simulink model "SDRE_MPTA_SDRE_newMODEL"  (R2024a)
settings: Solver=ode23t  StartTime=0  StopTime=27.8  RelTol=1e-3
values from neighbouring files (symbols this model uses):
  B = 0.002277    [initial_value.m]
  coef = readmatrix(ReadPath_coef)    [inital.m]
  command_t = readmatrix(ReadPath_command_t)    [inital.m]
  J = 0.00782    [initial_value.m]
  Lambda_m = 0.30175    [initial_value.m]
  Ld = 18e-3    (= 0.018)    [initial_value.m]
  Ldq = Ld - Lq    [inital.m]
  Lq = 32e-3    (= 0.032)    [initial_value.m]
  Polepairs = 3    [initial_value.m]
  rate1 = 3    [inital.m]
  rate2 = 1    [inital.m]
  Rs = 2.5    [initial_value.m]
  timestep = 1e-5    (= 1e-05)    [inital.m]
  V = [V_11 V_12;V_21 V_22]    [Create_MVG.m]
undefined symbols (not defined in the file or in its folder): rate
libraries: spsControlledVoltageSourceLib x6, spsPermanentMagnetSynchronousMachineLib x2, spsGroundLib x2, sps_lib x1
(part 2 of 2)

== matlab function SDRE_MPTA_SDRE_newMODEL/nomal3/toq to voltageABC6/MATLAB Function1 ==
  data: velo_fb input; id_fb input; iq_fb input; velo_ref input; id_ref input; iq_ref input; ud output; uq output; ud1 output; uq1 output; id_dot input; iq_dot input; ud2 output; uq2 output; velo_error output; id_error output; iq_error output
function [ud,uq,ud1,uq1,ud2,uq2,velo_error,id_error,iq_error] = SDRE_motor(velo_fb,id_fb,iq_fb,velo_ref,id_ref,iq_ref,id_dot,iq_dot)

ud = zeros(1, 1, 'double');
uq = zeros(1, 1, 'double');

%change data from [1*1] to singal input
Q = zeros(3, 3, 'double');

if isempty(id_dot)
    id_dot=0;
    iq_dot=0;
end


% velo_error   = 0;
% id_error     = 0;
% iq_error     = 0;

velo_error   = velo_fb   - velo_ref;
id_error     = id_fb     - id_ref;
iq_error     = iq_fb     - iq_ref;

if isempty(iq_error)
    velo_error=0;
    id_error=0;
    iq_error =0;
end

error = [velo_error iq_error id_error];

[Ld,Lq,Rs,Lambda_m,Polepairs,J,B]  = initial_value;
Ldq = Ld-Lq;

% A11 = -B/J; A12 = 3*Polepairs^2 *Lambda_m/(8*J); A13 = 3*Polepairs^2 *Ldq*iq_error/(8*J);
% A21 = -Lambda_m/(Lq) - Ld*id_error/(2*Lq); A22 = -Rs/Lq; A23 = - Ld*velo_error/(2*Lq);
% A31 = Lq*iq_error/(2*Ld); A32 =Lq*velo_error/(2*Ld); A33 = -Rs/Ld;

% A11 = -B/J; A12 = 3*Polepairs^2 *Lambda_m/(4*J); A13 = 3*Polepairs^2 *Ldq*iq_error/(4*J);
% A21 = -Lambda_m/(Lq) - Ld*id_error/(Lq); A22 = -Rs/Lq; A23 = 0;
% A31 = Lq*iq_error/(Ld); A32 =0; A33 = -Rs/Ld;
% 
% B11 = 0;B12 =0;
% B21=1/Lq;B22=0;
% B31=0;B32=1/Ld;

A11 = -B*Polepairs/J; A12 = 3*Polepairs^2 *(Lambda_m + Ldq*id_ref)/(2*J); A13 = 3*Polepairs^2 *Ldq*iq_fb/(2*J);
A21 = (-Lambda_m-Ld*id_fb)/(Lq) - Ld*id_error/(Lq); A22 = -Rs/Lq; A23 = -Ld*velo_ref/Lq;
A31 = Lq*iq_fb/(Ld); A32 =Lq*velo_ref/Ld; A33 = -Rs/Ld;

B11 = 0;B12 =0;
B21=1/Lq;B22=0;
B31=0;B32=1/Ld;


A = [A11 A12 A13 ;
     A21 A22 A23 ;
     A31 A32 A33];

B = [B11 B12;
     B21 B22;
     B31 B32];


rate = sqrt(iq_error^2 + id_error^2);
Q=diag([5000 1+exp(-rate) 10000+exp(-rate)]);
%Q=diag([800 1+exp(-rate) 100+exp(-rate)]);
R=diag([1 1]);

[P_ss_care,~]=SDA_CARE(A,B,Q,R);


% ucq = Rs*iq_ref + Lq*iq_dot + velo_ref*(Ld*id_ref+Lambda_m);
% ucd = Rs*id_ref + Ld*id_dot - velo_ref*Lq*iq_ref;


ucq = Rs*iq_ref + Lambda_m*velo_ref + Lq*iq_dot + Ld*id_error*velo_ref + Ld*velo_fb*id_ref;
ucd = Rs*id_ref + Ld*id_dot - Lq*iq_error*velo_ref - Lq*velo_fb*iq_ref;
if ucq > 1e5
    ucq =0;
end

if ucd > 1e5
    ucd =0;
end

u_redeem = -inv(R)*B'*P_ss_care*error';

% uq =  ucq ;
% ud =  ucd ;

uq =  ucq + u_redeem(1) ;
ud =  ucd + u_redeem(2) ;

ud1 = ucd ;
uq1 = ucq;

ud2 = u_redeem(2) ;
uq2 = u_redeem(1) ;


ud = (reshape(ud, 1, 1));
uq = (reshape(uq, 1, 1));


end

== matlab function SDRE_MPTA_SDRE_newMODEL/SDRE1 ==
  data: output_u1 output; Velocity1_ref output; T_load_1 output; Theta1_fb input; Velocity1_fb input; Acc1_fb input; Theta1_ref input; Theta3_ref input; Velocity1_ref input; Velocity3_ref input; Acc1_ref input; Acc3_ref input; output_u2 output; Velocity3_ref output; T_load_2 output; Theta3_fb input; Velocity3_fb input; Acc3_fb input; time input
function [output_u1,Velocity1_ref,T_load_1,output_u2,Velocity3_ref,T_load_2] = Robots_state(Theta1_fb,Velocity1_fb,Acc1_fb,Theta1_ref,Theta3_ref,Velocity1_ref,Velocity3_ref,Acc1_ref,Acc3_ref, Theta3_fb,  Velocity3_fb,Acc3_fb,time)
    %change data from [1*1] to singal input
    Acc3_ref = reshape(Acc3_ref, 1, []);

    Theta1_error =Theta1_fb - Theta1_ref;
    Velocity1_error = Velocity1_fb - Velocity1_ref;
    Acc1_error = Acc1_ref - Acc1_fb;

    Theta3_error = Theta3_fb - Theta3_ref;    
    Velocity3_error = Velocity3_fb - Velocity3_ref;
    Acc3_error = Acc3_ref - Acc3_fb;

    
    Acc_ref = [Acc1_ref;Acc3_ref];
    Velo_ref = [Velocity1_ref;Velocity3_ref];
    Theta_ref = [Theta1_ref;Theta3_ref];
    error_robot = [Theta1_error Theta3_error Velocity1_error Velocity3_error 0];

    Q=diag([10 10 1000 1000 0]);
    R=diag([1 1]);

    zeta = exp(-5*time);

    [M_fb,V_fb,G_sd_fb]=Create_MVG(Theta1_fb,Theta3_fb,Velocity1_fb,Velocity3_fb);
    [M_ref,V_ref,G_sd_ref]=Create_MVG(Theta1_ref,Theta3_ref,Velocity1_ref,Velocity3_ref);
    gf = M_fb*Acc_ref - M_ref*Acc_ref + V_fb*Velo_ref - V_ref*Velo_ref + G_sd_fb*Theta_ref - G_sd_ref*Theta_ref;
    A11 = zeros(2);
    A12 = eye(2);
    A13 = [0;0];
    A21 = -(M_fb)\G_sd_fb;
    A22 = -(M_fb)\V_fb;
    A23 = -((M_fb)\gf)/zeta;
    A31 = [0 0];
    A32 = [0 0];
    A33 = -5;
    A = [A11 A12 A13;A21 A22 A23;A31 A32 A33];
    B1 = zeros(2);
    B2 = inv(M_fb);
    B = [B1;B2;0 0];

    [P_ss_care,~]=SDA_CARE(A,B,Q,R);
    
    u1 = -inv(R)*B'*P_ss_care*error_robot';
    u_f1_1 = M_ref*[Acc1_ref Acc3_ref]';
    u_f1_2 = V_ref*[Velocity1_ref Velocity3_ref]';
    u_f1_3 = G_sd_ref*[Theta1_ref Theta3_ref]';
    u_f1 =  u_f1_1 + u_f1_2 + u_f1_3;

    output_u1 = u1(1) + u_f1(1);
    output_u2 = u1(2) + u_f1(2);

    [Ld,Lq,Rs,Lambda_m,Polepairs,J,B] = initial_value;
    ul_f1_1 = M_fb*[Acc1_fb Acc3_fb]';
    ul_f1_2 = V_fb*[Velocity1_fb Velocity3_fb]';
    ul_f1_3 = G_sd_fb*[Theta1_fb Theta3_fb]';
    ul_f1 =  ul_f1_1 + ul_f1_2 + ul_f1_3;
    % T_load_1 = ul_f1(1) ;
    % T_load_2 = ul_f1(2) ;
    display1 = ul_f1(1) ;
    display2 = ul_f1(2) ;   
    % 
    T_load_1 = u_f1(1) - J*Acc1_fb - B*Velocity1_fb - J*Acc1_error - B*Velocity1_error;
    T_load_2 = u_f1(2) - J*Acc3_fb - B*Velocity3_fb - J*Acc3_error - B*Velocity3_error;


    % output_u1 = (u1(1) + u_f1(1)) - T_load_1;
    % output_u2 = (u1(2) + u_f1(2)) - T_load_2 ;

    
end

== matlab function SDRE_MPTA_SDRE_newMODEL/target path input1/Subsystem1/Path function ==
  data: time input; Place output; Velocity output; Acc output
function [Place,Velocity,Acc] = fcn(time)



Place = (time^3)/4 *pi;
Velocity = 3/4 * time^2 *pi*10;
Acc = 3/2 * time * pi*10^2;


end

== matlab function SDRE_MPTA_SDRE_newMODEL/target path input1/Subsystem2/Path function ==
  data: time input; Place output; Velocity output; Acc output
function [Place,Velocity,Acc] = fcn(time)



% Place = time^3 /4 *pi;
% Velocity = 3/4 * time^2 *pi;
% Acc = 3/2 * time * pi;

Place = time^3 /4 *pi;
Velocity = 3/4 * time^2 *pi*10;
Acc = 3/2 * time * pi*10^2;

end

== matlab function SDRE_MPTA_SDRE_newMODEL/nomal1/toq to voltageABC6/MATLAB Function1 ==
  data: velo_fb input; id_fb input; iq_fb input; velo_ref input; id_ref input; iq_ref input; ud output; uq output; ud1 output; uq1 output; id_dot input; iq_dot input; ud2 output; uq2 output; velo_error output; id_error output; iq_error output
function [ud,uq,ud1,uq1,ud2,uq2,velo_error,id_error,iq_error] = SDRE_motor(velo_fb,id_fb,iq_fb,velo_ref,id_ref,iq_ref,id_dot,iq_dot)

ud = zeros(1, 1, 'double');
uq = zeros(1, 1, 'double');

%change data from [1*1] to singal input
Q = zeros(3, 3, 'double');

if isempty(id_dot)
    id_dot=0;
    iq_dot=0;
end


% velo_error   = 0;
% id_error     = 0;
% iq_error     = 0;

velo_error   = velo_fb   - velo_ref;
id_error     = id_fb     - id_ref;
iq_error     = iq_fb     - iq_ref;

if isempty(iq_error)
    velo_error=0;
    id_error=0;
    iq_error =0;
end

error = [velo_error iq_error id_error];

[Ld,Lq,Rs,Lambda_m,Polepairs,J,B]  = initial_value;
Ldq = Ld-Lq;

% A11 = -B/J; A12 = 3*Polepairs^2 *Lambda_m/(8*J); A13 = 3*Polepairs^2 *Ldq*iq_error/(8*J);
% A21 = -Lambda_m/(Lq) - Ld*id_error/(2*Lq); A22 = -Rs/Lq; A23 = - Ld*velo_error/(2*Lq);
% A31 = Lq*iq_error/(2*Ld); A32 =Lq*velo_error/(2*Ld); A33 = -Rs/Ld;

% A11 = -B/J; A12 = 3*Polepairs^2 *Lambda_m/(4*J); A13 = 3*Polepairs^2 *Ldq*iq_error/(4*J);
% A21 = -Lambda_m/(Lq) - Ld*id_error/(Lq); A22 = -Rs/Lq; A23 = 0;
% A31 = Lq*iq_error/(Ld); A32 =0; A33 = -Rs/Ld;
% 
% B11 = 0;B12 =0;
% B21=1/Lq;B22=0;
% B31=0;B32=1/Ld;

A11 = -B*Polepairs/J; A12 = 3*Polepairs^2 *(Lambda_m + Ldq*id_ref)/(2*J); A13 = 3*Polepairs^2 *Ldq*iq_fb/(2*J);
A21 = (-Lambda_m-Ld*id_fb)/(Lq) - Ld*id_error/(Lq); A22 = -Rs/Lq; A23 = -Ld*velo_ref/Lq;
A31 = Lq*iq_fb/(Ld); A32 =Lq*velo_ref/Ld; A33 = -Rs/Ld;

B11 = 0;B12 =0;
B21=1/Lq;B22=0;
B31=0;B32=1/Ld;


A = [A11 A12 A13 ;
     A21 A22 A23 ;
     A31 A32 A33];

B = [B11 B12;
     B21 B22;
     B31 B32];


rate = sqrt(iq_error^2 + id_error^2);
Q=diag([5000 1+exp(-rate) 10000+exp(-rate)]);
%Q=diag([800 1+exp(-rate) 100+exp(-rate)]);
R=diag([1 1]);

[P_ss_care,~]=SDA_CARE(A,B,Q,R);


% ucq = Rs*iq_ref + Lq*iq_dot + velo_ref*(Ld*id_ref+Lambda_m);
% ucd = Rs*id_ref + Ld*id_dot - velo_ref*Lq*iq_ref;


ucq = Rs*iq_ref + Lambda_m*velo_ref + Lq*iq_dot + Ld*id_error*velo_ref + Ld*velo_fb*id_ref;
ucd = Rs*id_ref + Ld*id_dot - Lq*iq_error*velo_ref - Lq*velo_fb*iq_ref;
if ucq > 1e5
    ucq =0;
end

if ucd > 1e5
    ucd =0;
end

u_redeem = -inv(R)*B'*P_ss_care*error';

% uq =  ucq ;
% ud =  ucd ;

uq =  ucq + u_redeem(1) ;
ud =  ucd + u_redeem(2) ;

ud1 = ucd ;
uq1 = ucq;

ud2 = u_redeem(2) ;
uq2 = u_redeem(1) ;


ud = (reshape(ud, 1, 1));
uq = (reshape(uq, 1, 1));


end

== matlab function SDRE_MPTA_SDRE_newMODEL/nomal1/MTPA ==
  data: id_ref output; Te input; iq_ref output
function [id_ref , iq_ref] = fcn(Te)

[Ld,Lq,Rs,Lambda_m,Polepairs,J,B]  = initial_value;
Ldq = Ld-Lq;

p1 = 3*Polepairs*Ldq^2 /(Lambda_m*2);
p2 = 0;
p3 = 3*Polepairs*Lambda_m/2;
p4 = -Te;
p = [p1 p2 p3 p4];
r = roots(p);

real_solutions = r(imag(r) == 0);


iq_ref = real(max(real_solutions));
id_ref = Ldq*iq_ref^2 /Lambda_m;

end

== matlab function SDRE_MPTA_SDRE_newMODEL/target path input1/MATLAB Function ==
  data: time input; Theta1_input output; velocity1_input output; acc1_input output; coef input; command_t input
function [Theta1_input,velocity1_input,acc1_input] = fcn(time,coef,command_t)
%total time 27.8
time = time/60;
l = length(command_t);
mode =1;
for i=1:l
    if time > command_t(i)
        mode = i;
    end
end


a_place=4*(mode-1); 
part_1_D = coef(a_place+1);
part_2_D = coef(a_place+2)*time;
part_3_D = coef(a_place+3)*time^2;
part_4_D  = coef(a_place+4)*time^3;

part_2_V = coef(a_place+2);
part_3_V = 2*coef(a_place+3)*time;   
part_4_V = 3*coef(a_place+4)*time^2;

part_3_A = 2*coef(a_place+3);  
part_4_A = 6*coef(a_place+4)*time;

Theta1_input = (part_1_D+part_2_D +part_3_D+part_4_D)*2*pi;
velocity1_input = (part_2_V + part_3_V + part_4_V)*2*pi/60;
acc1_input = (part_3_A+part_4_A)*2*pi/360;

% Theta1_input = 0;
% velocity1_input = 0;
% acc1_input = 0;

== matlab function SDRE_MPTA_SDRE_newMODEL/target path input1/MATLAB Function1 ==
  data: time input; Theta3_input output; velocity3_input output; acc3_input output; coef input; command_t input
function [Theta3_input,velocity3_input,acc3_input] = fcn(time,coef,command_t)
%total time 27.8
time = time/60;
l = length(command_t);
mode =1;
for i=1:l
    if time > command_t(i)
        mode = i;
    end
end


a_place=4*(mode-1); 
part_1_D = coef(a_place+1);
part_2_D = coef(a_place+2)*time;
part_3_D = coef(a_place+3)*time^2;
part_4_D  = coef(a_place+4)*time^3;

part_2_V = coef(a_place+2);
part_3_V = 2*coef(a_place+3)*time;   
part_4_V = 3*coef(a_place+4)*time^2;

part_3_A = 2*coef(a_place+3);  
part_4_A = 6*coef(a_place+4)*time;

Theta3_input = (part_1_D+part_2_D +part_3_D+part_4_D)*2*pi/7;
velocity3_input = (part_2_V + part_3_V + part_4_V)*2*pi/(60*7);
acc3_input = (part_3_A+part_4_A)*2*pi/(360*7);

% Theta3_input = 0;
% velocity3_input = 0;
% acc3_input = 0;

== matlab function SDRE_MPTA_SDRE_newMODEL/nomal3/MTPA ==
  data: id_ref output; Te input; iq_ref output
function [id_ref , iq_ref] = fcn(Te)

[Ld,Lq,Rs,Lambda_m,Polepairs,J,B]  = initial_value;
Ldq = Ld-Lq;

p1 = 3*Polepairs*Ldq^2 /(Lambda_m*2);
p2 = 0;
p3 = 3*Polepairs*Lambda_m/2;
p4 = -Te;
p = [p1 p2 p3 p4];
r = roots(p);

real_solutions = r(imag(r) == 0);


iq_ref = real(max(real_solutions));
id_ref = Ldq*iq_ref^2 /Lambda_m;
end
